simulink model "mpc_trace_Nurburgring"  (R2022b)
settings: Solver=ode45  StartTime=0.0  StopTime=30  FixedStep=0.01  RelTol=1e-3  EnableMultiTasking=on
libraries: Solver_SF x1
settings Model: Creator=xuwei  LastModifiedBy=wyx
settings SolverCC: AlgebraicLoopSolver=TrustRegion
settings DataIOCC: LimitDataPoints=on  SaveFormat=Array  SignalLoggingSaveFormat=ModelDataLogs  ReturnWorkspaceOutputs=off
settings OptimizationCC: ExpressionDepthLimit=2147483647  LifeSpan=inf
settings DebuggingCC: UnderspecifiedInitializationDetection=Classic  MergeDetectMultiDrivingBlocksExec=none  SolverPrmCheckMsg=warning  FcnCallInpInsideContextMsg=warning  UnconnectedInputMsg=warning  UnconnectedOutputMsg=warning  UnconnectedLineMsg=warning  StateNameClashWarn=warning  SFUnexpectedBacktrackingDiag=warning  SFNoUnconditionalDefaultTransitionDiag=warning  SFExecutionAtInitializationDiag=none  SFMachineParentedDataDiag=warning  ArithmeticOperatorsInVariantConditions=warning
settings HardwareCC: ProdBitPerPointer=32  ProdBitPerSizeT=32  ProdBitPerPtrDiffT=32  ProdLargestAtomicFloat=None  ProdIntDivRoundTo=Undefined  ProdEndianess=Unspecified  ProdWordSize=32  ProdHWDeviceType=32-bit Generic
settings ModelReferenceCC: PropagateSignalLabelsOutOfModel=off
settings SFSimCC: SimUseLocalCustomCode=off  CustomCodeUndefinedFunction=UseInterfaceOnly
settings RTWCC: RTWUseLocalCustomCode=off
settings CodeAppCC: StateflowObjectComments=on
settings GRTTargetCC: TargetLangStandard=C89/C90 (ANSI)  CombineOutputUpdateFcns=off  GRTInterface=on
settings ConfigComp: CovMetricSettings=dw  CovSaveCumulativeToWorkspaceVar=on  CovSaveSingleToWorkspaceVar=on  CovExternalEMLEnable=off
settings SimscapeCC: SimscapeNormalizeSystem=off
settings ConfigurationSet: Description=SimMechanics 2G

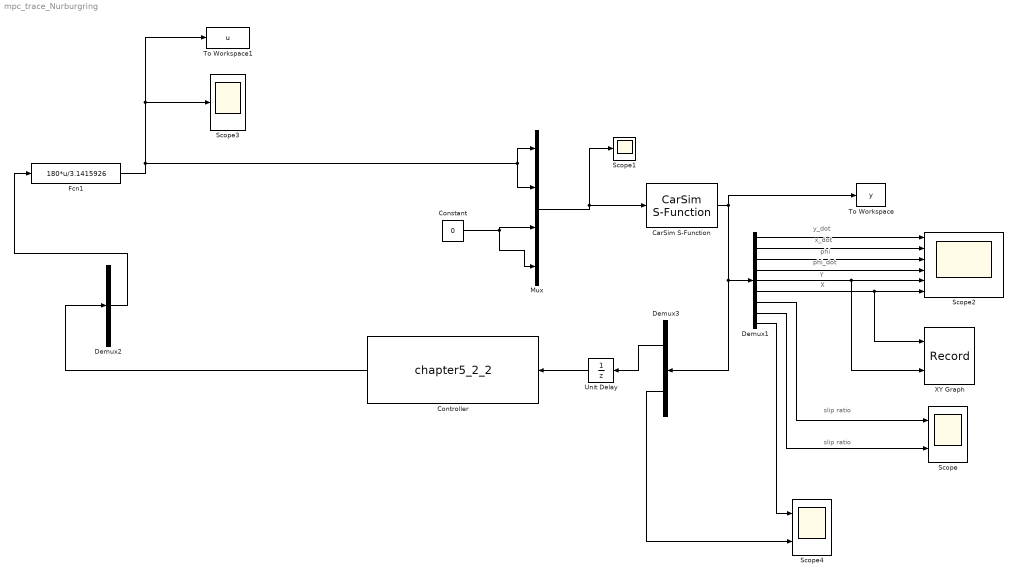
== system mpc_trace_Nurburgring ==
  note: y_dot
  note: x_dot
  note: phi
  note: phi_dot
  note: Y
  note: X
  note: slip ratio
  note: slip ratio
  CarSim S-Function : Solver_SF/CarSim S-Function  Priority=1  SIMFILE=simfile.sim
  Constant : Constant  Value=0
  Controller : S-Function  FunctionName=chapter5_2_2  SFunctionDeploymentMode=off  EnableBusSupport=off
  Demux1 : Demux  Outputs=9
  Demux2 : Demux  Outputs=1
  Demux3 : Demux  Outputs=2
  Fcn1 : Fcn  Expr=180*u/3.1415926
  Mux : Mux
  Scope : Scope  NumInputPorts=2
  Scope1 : Scope
  Scope2 : Scope  NumInputPorts=6
  Scope3 : Scope
  Scope4 : Scope  NumInputPorts=2
  To Workspace : ToWorkspace  VariableName=y  SaveFormat=Structure  SampleTime=-1
  To Workspace1 : ToWorkspace  VariableName=u  SaveFormat=Structure  SampleTime=-1
  Unit Delay : UnitDelay  SampleTime=-1  HasFrameUpgradeWarning=on
  XY Graph : Record  FileSettingsInternal="{\"entries\":[{\"content\":{\"excelSettings\":{\"content\":{},\"type\":\"Streamout.ExcelSettings\"}},\"type\":\"Streamout.FileSettingStorage\",\"uuid\":\"064649f1-00f1-4687-a007-5003d75545ce\"}],\"packageUris\":[\"http://schema.mathworks.com/mf0/streamout_blocks/R2020a\"],\"version\":\"1.0\"}"  Layout=[1 1]  SignalsInternal="{\"entries\":[{\"content\":{\"signals\":[{\"content\":{\"blockPath\":[\"chapter5/XY Graph\"],\"channel\":[],\"dimensions\":[1],\"domain\":\"chapter5/XY Graph\",\"lineColor\":\"#a2142f\",\"plots\":[1],\"port\":1,\"sid\":[\"\"],\"signalID\":1831,\"signalName\":\"Demux1:6\"},\"type\":\"RecordBlkView.Signal\",\"uuid\":\"cf936162-c5fb-4b6d-aaa3-7a1cd7854166\"},{\"content\":{\"blockPath\":[\"chapter5/XY Graph\"],\"channel\":[],\"dimensions\":[1],\"domain\":\"chapter5/XY Graph\",\"lineColor\":\"#139fff\",\"plots\":[1],\"port\":2,\"sid\":[\"\"],\"signalID\":1835,\"signalName\":\"Demux1:5\"},\"type\":\"RecordBlkView.Signal\",\"uuid\":\"bea3a8d6-7814-445d-b9f6-e38a7d90713d\"}]},\"type\":\"RecordBlkView.InputSignals\",\"uuid\":\"9a7cd8a3-b3f6-4b95-9412-c378514d1520\"}],\"packageUris\":[\"http://schema.mathworks.com/mf0/streamout_blocks/R2020a\"],\"version\":\"1.0\"}"  VisualizationBindings="{\"xyplotplugin\":{\"info\":[{\"series\":[{\"bindingParametersList\":[{\"parameter\":\"X-Axis\",\"signalID\":1831,\"signalName\":\"Demux1:6\"},{\"parameter\":\"Y-Axis\",\"signalID\":1835,\"signalName\":\"Demux1:5\"}],\"seriesID\":19408}],\"subplotID\":1}]}}"  CompatibilityTag=XY  st=-1
  wires:
  CarSim S-Function/1 -> To Workspace/1, Demux3/1, Demux1/1
  Demux1/1 -> Scope2/1
  Demux1/2 -> Scope2/2
  Demux1/3 -> Scope2/3
  Demux1/4 -> Scope2/4
  Demux1/5 -> XY Graph/2, Scope2/5
  Demux1/6 -> XY Graph/1, Scope2/6
  Unit Delay/1 -> Controller/1
  Demux1/7 -> Scope/1
  Demux1/8 -> Scope/2
  Mux/1 -> Scope1/1, CarSim S-Function/1
  Controller/1 -> Demux2/1
  Constant/1 -> Mux/3, Mux/4
  Fcn1/1 -> Mux/1, Mux/2, Scope3/1, To Workspace1/1
  Demux2/1 -> Fcn1/1
  Demux1/9 -> Scope4/1
  Demux3/1 -> Unit Delay/1
  Demux3/2 -> Scope4/2
